simulink model "snap2_f_200msps_64i_4096c"  (R2019a)
settings: Solver=VariableStepDiscrete  StartTime=0.0  StopTime=10.0  RelTol=1e-3
undefined symbols (not defined in the file or in its folder): datetime, posixtime
libraries: xbsIndex_r4 x21354, casper_library_misc x297, casper_library_delays x19, xps_library x14, casper_library_sources x4
(part 2 of 217)

== system snap2_f_200msps_64i_4096c/SNAP2 ==

== system snap2_f_200msps_64i_4096c/aaa_onegbe ==
  Constant : xbsIndex_r4/Constant  const=0  gui_display_data_type=Boolean  arith_type=Boolean  n_bits=16  bin_pt=14  preci_type=Single  exp_width=8  frac_width=24  explicit_period=on  period=1  equ=P=C  opselect=C  inp2=PCIN>>17  opr=+  inp1=P  carry=CIN  dbl_ovrd=off  block_type=constant
  Constant1 : xbsIndex_r4/Constant  const=0  gui_display_data_type=Fixed-point  arith_type=Unsigned  n_bits=8  bin_pt=0  preci_type=Single  exp_width=8  frac_width=24  explicit_period=on  period=1  equ=P=C  opselect=C  inp2=PCIN>>17  opr=+  inp1=P  carry=CIN  dbl_ovrd=off  block_type=constant
  Constant2 : xbsIndex_r4/Constant  const=1  gui_display_data_type=Boolean  arith_type=Boolean  n_bits=16  bin_pt=14  preci_type=Single  exp_width=8  frac_width=24  explicit_period=on  period=1  equ=P=C  opselect=C  inp2=PCIN>>17  opr=+  inp1=P  carry=CIN  dbl_ovrd=off  block_type=constant
  Constant3 : xbsIndex_r4/Constant  const=0  gui_display_data_type=Fixed-point  arith_type=Unsigned  n_bits=32  bin_pt=0  preci_type=Single  exp_width=8  frac_width=24  explicit_period=on  period=1  equ=P=C  opselect=C  inp2=PCIN>>17  opr=+  inp1=P  carry=CIN  dbl_ovrd=off  block_type=constant
  Constant4 : xbsIndex_r4/Constant  const=0  gui_display_data_type=Fixed-point  arith_type=Unsigned  n_bits=16  bin_pt=0  preci_type=Single  exp_width=8  frac_width=24  explicit_period=on  period=1  equ=P=C  opselect=C  inp2=PCIN>>17  opr=+  inp1=P  carry=CIN  dbl_ovrd=off  block_type=constant
  one_GbE : xps_library/IO/one_gbe  Tag=xps:onegbe  local_en=on  dis_cpu_rx=off  dis_cpu_tx=off  cpu_promiscuous=off  local_mac=hex2dec('123456789abc')  local_ip=hex2dec('c0a8290a')  local_port=4321  local_gateway=1
      settings: SourceProductName=CASPER XPS Blockset
  wires:
  Constant/1 -> one_GbE/7, one_GbE/4, one_GbE/2, one_GbE/1
  Constant3/1 -> one_GbE/5
  Constant1/1 -> one_GbE/3
  Constant2/1 -> one_GbE/8
  Constant4/1 -> one_GbE/6

== system snap2_f_200msps_64i_4096c/adc ==
  chip_sync : Inport
  Delay{1..70,72} (71 alike) : xbsIndex_r4/Delay  rst=off  infoeditControl=Selection of Reset will increase slice count due to use of real FFs and instead of SRLs  en=off  latency=1  reg_retiming=off  dbl_ovrd=off  block_type=delay
  Logical : xbsIndex_r4/Logical  logical_function=OR  inputs=2  en=off  latency=1  precision=Full  arith_type=Unsigned  n_bits=16  bin_pt=0  align_bp=on  dbl_ovrd=off  block_type=logical
  Logical1 : xbsIndex_r4/Logical  logical_function=AND  inputs=2  en=off  latency=1  precision=Full  arith_type=Unsigned  n_bits=16  bin_pt=0  align_bp=on  dbl_ovrd=off  block_type=logical
  Logical3 : xbsIndex_r4/Logical  logical_function=OR  inputs=2  en=off  latency=1  precision=Full  arith_type=Unsigned  n_bits=16  bin_pt=0  align_bp=on  dbl_ovrd=off  block_type=logical
  Logical4 : xbsIndex_r4/Logical  logical_function=AND  inputs=2  en=off  latency=1  precision=Full  arith_type=Unsigned  n_bits=16  bin_pt=0  align_bp=on  dbl_ovrd=off  block_type=logical
  bus_create : Subsystem  AncestorBlock=casper_library_flow_control/bus_create  mask(bus_create){inputNum=64}
      mask prompts: inputNum "Number of inputs:"
      mask init:
      | bus_create_init(gcb,...
      |     'inputNum', inputNum);
  fmc0 : Subsystem  Tag=xps:ads5296x4  AncestorBlock=xps_library/ADCs/ads5296x4  mask(ADS5296x4){board_count=2, sample_rate=200, port=0, clockport=1, version=2}
      mask prompts: board_count "Number of quad-chip ADC Boards"; sample_rate "Sample Rate"; port "Which FMC port?"; clockport "Use clock from which FMC board?"; version "Which ADC board version?"
      mask help: 16-input ADC based on the TI ADS5296 chip.
      mask init:
      | % Only board_count is needed by init function
      | ads5296x4_init(gcb, ...
      |     'board_count', board_count);
      mask TypeOptions board_count: 1 | 2 | 3 | 4
  fmc1 : Subsystem  Tag=xps:ads5296x4  AncestorBlock=xps_library/ADCs/ads5296x4  mask(ADS5296x4){board_count=2, sample_rate=200, port=1, clockport=1, version=2}
      mask prompts: board_count "Number of quad-chip ADC Boards"; sample_rate "Sample Rate"; port "Which FMC port?"; clockport "Use clock from which FMC board?"; version "Which ADC board version?"
      mask help: 16-input ADC based on the TI ADS5296 chip.
      mask init:
      | % Only board_count is needed by init function
      | ads5296x4_init(gcb, ...
      |     'board_count', board_count);
      mask TypeOptions board_count: 1 | 2 | 3 | 4
  sync : Subsystem  Tag=xps:sw_reg  AncestorBlock=xps_library/Memory/software_register  mask(swreg){io_dir=From Processor, io_delay=0, init_val=0, sample_period=1, names=[sync ext_sync_enable ss_trig ext_ss_trig_en rst], bitwidths=[1 1 1 1 1], bin_pts=0, arith_types=2, sim_port=on, show_format=on, desc_str=|}
      mask desc_str=|
      | Write ``1`` to bit 0 to this register to assert the ADC's ``sync``
      | input. This input is edge sensitive.
      | Write ``1`` to bit 1 of this register to enable the external sync input.
      mask prompts: io_dir "I/O direction"; io_delay "I/O delay"; init_val "Initial Value"; sample_period "Sample period"; names "Bitfield names [msb...lsb]"; bitwidths "Bitfield widths"; bin_pts "Bitfield binary pts"; arith_types "Bitfield types, ufix=0, fix=1, bool=2"; sim_port "Provide sim input/output?"; show_format "Print format string?"; desc_str "Description"
      mask help: A 32-bit software-accessible register. Can be divided into bitfields of varying widths and types using the fields in the block mask.
      mask init:
      | swreg_init(gcb)
      settings: AttributesFormatString=5 inputs:b,b,b,b,b = 5 bits
      mask TypeOptions io_dir: To Processor | From Processor
      mask Callback io_dir:
      | mask_enables = get_param(gcb, 'MaskEnables');
      | mask_names = get_param(gcb, 'MaskNames');
      | if strcmp(get_param(gcb, 'io_dir'), 'To Processor'),
      |     mask_enables{ismember(mask_names, 'sample_period')} = 'off';
      | else
      |     mask_enables{ismember(mask_names, 'sample_period')} = 'on';
      | end
      | set_param(gcb, 'MaskEnables', mask_enables);
      mask DialogControl ParameterTabVar0 Prompt: Setup
  adc_data : Outport
  adc_sync : Outport  Port=2
  wires:
  fmc0/33(sync_out) -> ?
  bus_create/1(bus_out) -> adc_data/1
  Delay1/1 -> fmc1/33(sync)
  Delay2/1 -> fmc1/34(snapshot_trig)
  Delay3/1 -> fmc1/36(rst)
  Delay4/1 -> fmc0/36(rst)
  Delay5/1 -> fmc0/34(snapshot_trig)
  Delay6/1 -> fmc0/33(sync)
  fmc1/33(sync_out) -> Delay72/1
  Logical1/1 -> Logical/1
  sync/1(in_sync) -> [int_sync]
  sync/2(in_ext_sync_enable) -> [ext_sync_en]
  sync/3(in_ss_trig) -> [ss_trig]
  sync/4(in_ext_ss_trig_en) -> [ext_ss_trig_en]
  sync/5(in_rst) -> [rst]
  [rst] -> Delay4/1
  [rst] -> Delay3/1
  [ext_sync_en] -> Logical1/2
  [int_sync] -> Logical/2
  Logical/1 -> [adc_sync]
  [adc_sync] -> Delay6/1
  [adc_sync] -> Delay1/1
  Logical3/1 -> [adc_ss_trigger]
  [ss_trig] -> Logical3/2
  [ext_ss_trig_en] -> Logical4/2
  chip_sync/1 -> Logical4/1, Logical1/1
  Logical4/1 -> Logical3/1
  [adc_ss_trigger] -> Delay5/1
  [adc_ss_trigger] -> Delay2/1
  fmc0/1(a1) -> Delay7/1
  fmc0/2(a2) -> Delay8/1
  fmc0/3(a3) -> Delay9/1
  fmc0/4(a4) -> Delay10/1
  fmc0/5(b1) -> Delay12/1
  fmc0/6(b2) -> Delay13/1
  fmc0/7(b3) -> Delay14/1
  fmc0/8(b4) -> Delay11/1
  fmc0/9(c1) -> Delay20/1
  fmc0/10(c2) -> Delay21/1
  fmc0/11(c3) -> Delay22/1
  fmc0/12(c4) -> Delay15/1
  fmc0/13(d1) -> Delay17/1
  fmc0/14(d2) -> Delay18/1
  fmc0/15(d3) -> Delay19/1
  fmc0/19(e3) -> Delay38/1
  fmc0/20(e4) -> Delay23/1
  fmc0/22(f2) -> Delay26/1
  fmc0/26(g2) -> Delay34/1
  fmc0/30(h2) -> Delay31/1
  fmc0/25(g1) -> Delay33/1
  fmc0/23(f3) -> Delay27/1
  fmc0/18(e2) -> Delay37/1
  fmc0/24(f4) -> Delay24/1
  fmc0/28(g4) -> Delay28/1
  fmc0/16(d4) -> Delay16/1
  fmc0/27(g3) -> Delay35/1
  fmc0/17(e1) -> Delay36/1
  fmc0/21(f1) -> Delay25/1
  fmc0/29(h1) -> Delay30/1
  fmc1/25(g1) -> Delay65/1
  fmc1/2(a2) -> Delay53/1
  fmc1/10(c2) -> Delay50/1
  fmc1/5(b1) -> Delay41/1
  fmc1/4(a4) -> Delay39/1
  fmc1/12(c4) -> Delay44/1
  fmc1/7(b3) -> Delay43/1
  fmc1/18(e2) -> Delay69/1
  fmc1/22(f2) -> Delay58/1
  fmc1/14(d2) -> Delay47/1
  fmc1/19(e3) -> Delay70/1
  fmc1/17(e1) -> Delay68/1
  fmc1/1(a1) -> Delay52/1
  fmc1/24(f4) -> Delay56/1
  fmc0/31(h3) -> Delay32/1
  fmc1/27(g3) -> Delay67/1
  fmc1/8(b4) -> Delay40/1
  fmc1/15(d3) -> Delay48/1
  fmc1/11(c3) -> Delay51/1
  fmc1/13(d1) -> Delay46/1
  fmc0/32(h4) -> Delay29/1
  fmc1/6(b2) -> Delay42/1
  fmc1/3(a3) -> Delay54/1
  fmc1/16(d4) -> Delay45/1
  fmc1/26(g2) -> Delay66/1
  fmc1/9(c1) -> Delay49/1
  fmc1/21(f1) -> Delay57/1
  fmc1/23(f3) -> Delay59/1
  fmc1/20(e4) -> Delay55/1
  fmc1/28(g4) -> Delay60/1
  fmc1/32(h4) -> Delay61/1
  fmc1/30(h2) -> Delay63/1
  fmc1/31(h3) -> Delay64/1
  fmc1/29(h1) -> Delay62/1
  Delay72/1 -> adc_sync/1
  Delay7/1 -> bus_create/1(in1)
  Delay8/1 -> bus_create/2(in2)
  Delay9/1 -> bus_create/3(in3)
  Delay10/1 -> bus_create/4(in4)
  Delay13/1 -> bus_create/6(in6)
  Delay14/1 -> bus_create/7(in7)
  Delay12/1 -> bus_create/5(in5)
  Delay11/1 -> bus_create/8(in8)
  Delay21/1 -> bus_create/10(in10)
  Delay17/1 -> bus_create/13(in13)
  Delay16/1 -> bus_create/16(in16)
  Delay20/1 -> bus_create/9(in9)
  Delay15/1 -> bus_create/12(in12)
  Delay22/1 -> bus_create/11(in11)
  Delay19/1 -> bus_create/15(in15)
  Delay18/1 -> bus_create/14(in14)
  Delay26/1 -> bus_create/22(in22)
  Delay33/1 -> bus_create/25(in25)
  Delay35/1 -> bus_create/27(in27)
  Delay34/1 -> bus_create/26(in26)
  Delay36/1 -> bus_create/17(in17)
  Delay27/1 -> bus_create/23(in23)
  Delay32/1 -> bus_create/31(in31)
  Delay25/1 -> bus_create/21(in21)
  Delay29/1 -> bus_create/32(in32)
  Delay38/1 -> bus_create/19(in19)
  Delay28/1 -> bus_create/28(in28)
  Delay31/1 -> bus_create/30(in30)
  Delay30/1 -> bus_create/29(in29)
  Delay24/1 -> bus_create/24(in24)
  Delay37/1 -> bus_create/18(in18)
  Delay23/1 -> bus_create/20(in20)
  Delay42/1 -> bus_create/38(in38)
  Delay50/1 -> bus_create/42(in42)
  Delay39/1 -> bus_create/36(in36)
  Delay53/1 -> bus_create/34(in34)
  Delay51/1 -> bus_create/43(in43)
  Delay40/1 -> bus_create/40(in40)
  Delay52/1 -> bus_create/33(in33)
  Delay47/1 -> bus_create/46(in46)
  Delay41/1 -> bus_create/37(in37)
  Delay54/1 -> bus_create/35(in35)
  Delay49/1 -> bus_create/41(in41)
  Delay43/1 -> bus_create/39(in39)
  Delay48/1 -> bus_create/47(in47)
  Delay44/1 -> bus_create/44(in44)
  Delay46/1 -> bus_create/45(in45)
  Delay45/1 -> bus_create/48(in48)
  Delay55/1 -> bus_create/52(in52)
  Delay60/1 -> bus_create/60(in60)
  Delay65/1 -> bus_create/57(in57)
  Delay68/1 -> bus_create/49(in49)
  Delay66/1 -> bus_create/58(in58)
  Delay69/1 -> bus_create/50(in50)
  Delay64/1 -> bus_create/63(in63)
  Delay56/1 -> bus_create/56(in56)
  Delay58/1 -> bus_create/54(in54)
  Delay59/1 -> bus_create/55(in55)
  Delay70/1 -> bus_create/51(in51)
  Delay62/1 -> bus_create/61(in61)
  Delay61/1 -> bus_create/64(in64)
  Delay57/1 -> bus_create/53(in53)
  Delay63/1 -> bus_create/62(in62)
  Delay67/1 -> bus_create/59(in59)

== system snap2_f_200msps_64i_4096c/autocorr ==
  note: acc_len in spectra
  sync : Inport
  din : Inport  Port=2
  rst : Inport  Port=3
  0 : Subsystem  Commented=on  mask{nchan_bits=nchan_bits, npol_bits=npol_bits - 2}
      mask prompts: nchan_bits "Number of channels (2^?)"; npol_bits "Number of pols (2^?)"
  1 : Subsystem  Commented=on  mask{nchan_bits=nchan_bits, npol_bits=npol_bits - 2}
      mask prompts: nchan_bits "Number of channels (2^?)"; npol_bits "Number of pols (2^?)"
  2 : Subsystem  Commented=on  mask{nchan_bits=nchan_bits, npol_bits=npol_bits - 2}
      mask prompts: nchan_bits "Number of channels (2^?)"; npol_bits "Number of pols (2^?)"
  3 : Subsystem  Commented=on  mask{nchan_bits=nchan_bits, npol_bits=npol_bits - 2}
      mask prompts: nchan_bits "Number of channels (2^?)"; npol_bits "Number of pols (2^?)"
  Constant : xbsIndex_r4/Constant  const=0  gui_display_data_type=Fixed-point  arith_type=Unsigned  n_bits=288  bin_pt=0  preci_type=Single  exp_width=8  frac_width=24  explicit_period=on  period=1  equ=P=C  opselect=C  inp2=PCIN>>17  opr=+  inp1=P  carry=CIN  dbl_ovrd=off  block_type=constant
  Constant6 : Constant  Value=1024
  Counter1 : xbsIndex_r4/Counter  cnt_type=Free Running  cnt_to=Inf  operation=Up  start_count=0  cnt_by_val=1  arith_type=Unsigned  n_bits=32  bin_pt=0  load_pin=off  rst=off  en=on  explicit_period=on  period=1  use_behavioral_HDL=off  implementation=Fabric  dbl_ovrd=off  block_type=counter
  Delay1 : xbsIndex_r4/Delay  rst=off  infoeditControl=Selection of Reset will increase slice count due to use of real FFs and instead of SRLs  en=off  latency=1  reg_retiming=on  dbl_ovrd=off  block_type=delay
  Delay2 : xbsIndex_r4/Delay  rst=off  infoeditControl=Selection of Reset will increase slice count due to use of real FFs and instead of SRLs  en=off  latency=1  reg_retiming=on  dbl_ovrd=off  block_type=delay
  Delay3 : xbsIndex_r4/Delay  rst=off  infoeditControl=Selection of Reset will increase slice count due to use of real FFs and instead of SRLs  en=off  latency=3  reg_retiming=on  dbl_ovrd=off  block_type=delay
  From{,2,5,10} (4 alike) : From  Commented=on  GotoTag=sync
  From{1,3,6,11} (4 alike) : From  Commented=on  GotoTag=rst
  From{4,7,9,12} (4 alike) : From  Commented=on  GotoTag=acc_len
  From13 : From  Commented=on  GotoTag=chan16_32
  From14 : From  Commented=on  GotoTag=chan32_48
  From15 : From  Commented=on  GotoTag=chan48_64
  From16 : From  Commented=on  GotoTag=chan0_16
  From{25..28} (4 alike) : From  Commented=on  GotoTag=trig
  Goto2 : Goto  Commented=on  GotoTag=new_acc
  Mux : xbsIndex_r4/Mux  inputs=5  en=off  latency=1  precision=Full  arith_type=Unsigned  n_bits=16  bin_pt=14  quantization=Truncate  overflow=Wrap  dbl_ovrd=off  block_type=mux
  Slice1 : xbsIndex_r4/Slice  nbits=32-nchan_bits-npol_bits  boolean_output=off  mode=Lower Bit Location + Width  bit1=0  base1=MSB of Input  bit0=0  base0=LSB of Input  dbl_ovrd=off  block_type=slice
  acc_cnt : Subsystem  Tag=xps:sw_reg  AncestorBlock=xps_library/Memory/software_register  mask(swreg){io_dir=To Processor, io_delay=0, init_val=0, sample_period=1, names=reg, bitwidths=32, bin_pts=0, arith_types=0, sim_port=on, show_format=on, desc_str=|}
      mask desc_str=|
      | 32-bit wrapping accumulation counter, which increments each
      | time a new accumulation is recorded to RAM.
      | There is no buffer locking when correlation data are
      | read, so this counter can be used to ensure that data
      | have not changed during a read.
      mask prompts: io_dir "I/O direction"; io_delay "I/O delay"; init_val "Initial Value"; sample_period "Sample period"; names "Bitfield names [msb...lsb]"; bitwidths "Bitfield widths"; bin_pts "Bitfield binary pts"; arith_types "Bitfield types, ufix=0, fix=1, bool=2"; sim_port "Provide sim input/output?"; show_format "Print format string?"; desc_str "Description"
      mask help: A 32-bit software-accessible register. Can be divided into bitfields of varying widths and types using the fields in the block mask.
      mask init:
      | swreg_init(gcb)
      settings: AttributesFormatString=1output:uf32.0 = 32 bits
      mask TypeOptions io_dir: To Processor | From Processor
      mask Callback io_dir:
      | mask_enables = get_param(gcb, 'MaskEnables');
      | mask_names = get_param(gcb, 'MaskNames');
      | if strcmp(get_param(gcb, 'io_dir'), 'To Processor'),
      |     mask_enables{ismember(mask_names, 'sample_period')} = 'off';
      | else
      |     mask_enables{ismember(mask_names, 'sample_period')} = 'on';
      | end
      | set_param(gcb, 'MaskEnables', mask_enables);
      mask DialogControl ParameterTabVar0 Prompt: Setup
  acc_len : Subsystem  Tag=xps:sw_reg  AncestorBlock=xps_library/Memory/software_register  mask(swreg){io_dir=From Processor, io_delay=0, init_val=0, sample_period=1, names=reg, bitwidths=32, bin_pts=0, arith_types=0, sim_port=on, show_format=on, desc_str=Accumulation length, in spectra.}
      mask prompts: io_dir "I/O direction"; io_delay "I/O delay"; init_val "Initial Value"; sample_period "Sample period"; names "Bitfield names [msb...lsb]"; bitwidths "Bitfield widths"; bin_pts "Bitfield binary pts"; arith_types "Bitfield types, ufix=0, fix=1, bool=2"; sim_port "Provide sim input/output?"; show_format "Print format string?"; desc_str "Description"
      mask help: A 32-bit software-accessible register. Can be divided into bitfields of varying widths and types using the fields in the block mask.
      mask init:
      | swreg_init(gcb)
      settings: AttributesFormatString=1input:uf32.0 = 32 bits
      mask TypeOptions io_dir: To Processor | From Processor
      mask Callback io_dir:
      | mask_enables = get_param(gcb, 'MaskEnables');
      | mask_names = get_param(gcb, 'MaskNames');
      | if strcmp(get_param(gcb, 'io_dir'), 'To Processor'),
      |     mask_enables{ismember(mask_names, 'sample_period')} = 'off';
      | else
      |     mask_enables{ismember(mask_names, 'sample_period')} = 'on';
      | end
      | set_param(gcb, 'MaskEnables', mask_enables);
      mask DialogControl ParameterTabVar0 Prompt: Setup
  bus_expand : Subsystem  AncestorBlock=casper_library_flow_control/bus_expand  mask(bus_expand){mode=divisions of equal size, outputNum=4, outputWidth=18*2*8, outputBinaryPt=0, outputArithmeticType=0, show_format=off, outputToWorkspace=off, variablePrefix=out, outputToModelAsWell=on}
      mask prompts: outputNum "Number of outputs:"; outputWidth "Output width:"; outputBinaryPt "Output binary point position:"; outputArithmeticType "Output arithmetic type (ufix=0, fix=1, bool=2):"; show_format "Print format string?"; outputToWorkspace "Output to workspace?"; variablePrefix "Variable name prefix:"; outputToModelAsWell "Output to model as well?"
      mask help:
      | Expands a 'bus' made using a bus_create or Xilinx
      | concat block.
      | The input will be divided into the specified number
      | of outputs with the specified arithmetic types.
      | Divisions are made from most significant bit.
      mask init:
      | bus_expand_init(gcb,...
      |     'mode', mode, ...
      |     'outputNum', outputNum, ...
      |     'outputWidth', outputWidth, ...
      |     'outputBinaryPt', outputBinaryPt, ...
      |     'outputArithmeticType', outputArithmeticType, ...
      |     'show_format', show_format, ...
      |     'outputToWorkspace', outputToWorkspace, ...
      |     'variablePrefix', variablePrefix, ...
      |     'outputToModelAsWell', outputToModelAsWell);
      settings: AttributesFormatString=4 outputs
      mask TypeOptions mode: divisions of equal size | divisions of arbitrary size
      mask Callback mode: bus_expand_callback();
      mask Callback outputWidth: bus_expand_callback();
      mask Callback outputToWorkspace: bus_expand_callback();
  common : Subsystem  mask{nchan_bits=nchan_bits, npol_bits=npol_bits - 2}
      mask prompts: nchan_bits "Number of channels (2^?)"; npol_bits "Number of pols (2^?)"
  mux_sel : Subsystem  Tag=xps:sw_reg  AncestorBlock=xps_library/Memory/software_register  mask(swreg){io_dir=From Processor, io_delay=0, init_val=0, sample_period=1, names=reg, bitwidths=3, bin_pts=0, arith_types=0, sim_port=on, show_format=on, desc_str=|}
      mask desc_str=|
      | Input selection controller. Set bits ``[1:0]`` to ``n``
      | to compute the autocorrelations of F-engine inputs
      | ``16n..16(n+1)-1``.
      mask prompts: io_dir "I/O direction"; io_delay "I/O delay"; init_val "Initial Value"; sample_period "Sample period"; names "Bitfield names [msb...lsb]"; bitwidths "Bitfield widths"; bin_pts "Bitfield binary pts"; arith_types "Bitfield types, ufix=0, fix=1, bool=2"; sim_port "Provide sim input/output?"; show_format "Print format string?"; desc_str "Description"
      mask help: A 32-bit software-accessible register. Can be divided into bitfields of varying widths and types using the fields in the block mask.
      mask init:
      | swreg_init(gcb)
      settings: AttributesFormatString=1input:uf3.0 = 3 bits
      mask TypeOptions io_dir: To Processor | From Processor
      mask Callback io_dir:
      | mask_enables = get_param(gcb, 'MaskEnables');
      | mask_names = get_param(gcb, 'MaskNames');
      | if strcmp(get_param(gcb, 'io_dir'), 'To Processor'),
      |     mask_enables{ismember(mask_names, 'sample_period')} = 'off';
      | else
      |     mask_enables{ismember(mask_names, 'sample_period')} = 'on';
      | end
      | set_param(gcb, 'MaskEnables', mask_enables);
      mask DialogControl ParameterTabVar0 Prompt: Setup
  trig : Subsystem  Tag=xps:sw_reg  AncestorBlock=xps_library/Memory/software_register  mask(swreg){io_dir=From Processor, io_delay=0, init_val=0, sample_period=1, names=reg, bitwidths=1, bin_pts=0, arith_types=2, sim_port=on, show_format=on, desc_str="Transition bit 0 from 0 to 1 to trigger a capture of the next valid accumulation"}
      mask prompts: io_dir "I/O direction"; io_delay "I/O delay"; init_val "Initial Value"; sample_period "Sample period"; names "Bitfield names [msb...lsb]"; bitwidths "Bitfield widths"; bin_pts "Bitfield binary pts"; arith_types "Bitfield types, ufix=0, fix=1, bool=2"; sim_port "Provide sim input/output?"; show_format "Print format string?"; desc_str "Description"
      mask help: A 32-bit software-accessible register. Can be divided into bitfields of varying widths and types using the fields in the block mask.
      mask init:
      | swreg_init(gcb)
      settings: AttributesFormatString=1input:b = 1 bits
      mask TypeOptions io_dir: To Processor | From Processor
      mask Callback io_dir:
      | mask_enables = get_param(gcb, 'MaskEnables');
      | mask_names = get_param(gcb, 'MaskNames');
      | if strcmp(get_param(gcb, 'io_dir'), 'To Processor'),
      |     mask_enables{ismember(mask_names, 'sample_period')} = 'off';
      | else
      |     mask_enables{ismember(mask_names, 'sample_period')} = 'on';
      | end
      | set_param(gcb, 'MaskEnables', mask_enables);
      mask DialogControl ParameterTabVar0 Prompt: Setup
  wires:
  din/1 -> bus_expand/1(bus_in)
  sync/1 -> [sync]
  rst/1 -> [rst]
  From/1 -> 0/1(sync)
  From1/1 -> 0/3(rst)
  acc_len/1(in_reg) -> Slice1/1
  Constant6/1 -> acc_len/1(sim_1)
  Slice1/1 -> [acc_len]
  [new_acc] -> Counter1/1
  Delay2/1 -> acc_cnt/1(out_reg)
  Counter1/1 -> Delay2/1
  From9/1 -> 0/4(acc_len)
  From4/1 -> 1/4(acc_len)
  From3/1 -> 1/3(rst)
  From2/1 -> 1/1(sync)
  From5/1 -> 2/1(sync)
  From6/1 -> 2/3(rst)
  From7/1 -> 2/4(acc_len)
  From12/1 -> 3/4(acc_len)
  From11/1 -> 3/3(rst)
  From10/1 -> 3/1(sync)
  bus_expand/1(msb_out4) -> [chan0_16]
  bus_expand/2(out3) -> [chan16_32]
  bus_expand/3(out2) -> [chan32_48]
  bus_expand/4(lsb_out1) -> [chan48_64]
  From13/1 -> 1/2(din)
  From14/1 -> 2/2(din)
  From15/1 -> 3/2(din)
  From16/1 -> 0/2(din)
  Mux/1 -> common/2(din)
  [acc_len] -> common/4(acc_len)
  common/1(new_acc) -> [new_acc]
  [rst] -> common/3(rst)
  [sync] -> Delay1/1
  Delay1/1 -> common/1(sync)
  [chan0_16] -> Mux/2
  mux_sel/1(in_reg) -> Delay3/1
  [chan16_32] -> Mux/3
  [chan32_48] -> Mux/4
  [chan48_64] -> Mux/5
  Delay3/1 -> Mux/1
  [trig] -> common/5(trig)
  trig/1(in_reg) -> [trig]
  From25/1 -> 0/5(trig)
  0/1(new_acc) -> Goto2/1
  From26/1 -> 1/5(trig)
  From27/1 -> 2/5(trig)
  From28/1 -> 3/5(trig)
  Constant/1 -> Mux/6

== system snap2_f_200msps_64i_4096c/chan_reorder ==
  note: manually make
      | runtime configurable
      |
      | NB: allowed sync period
      | is unknown!!
  note: block transpose
      | last two words, so pol order is
      | 0, 1, ..., 31 (first word)
      | 32, 33, ..., 63 (second word)
  note: blockwise transpose:
      |
      | output order is now:
      |
      | chans (512) x pols (2) x chans (8) x pols (32)
      |
      | last axis here is pol:
      | n, n+16, n+32, n+48,
      | n+1, n+17, n+32, n+49, ...
      | ...
      | n+7, n+23, n+39, n+55
  note: Reorder each word:
      |
      | order is now:
      |
      | chans (512) x pols (16) x chans (8) x pols (4)
      |
      | Last index here is pol: n, n+16, n+32, n+48
  note: Input order is:
      |
      | pols (16) x chans (512) x pols (4) x chans (8)
      |
      | Transpose first two axes. Output order is:
      | chans (512) x pols (16) x pols (4) x chans (8)
  note: Use this programmable
      | map to mess with the channel
      | ordering.
      |
      | Out of every block of 128 channels,
      | only the first 80 will be sent.
      | So fold the edges of the band into unwanted slots
      |
      | Input is 8 channels x 4 antennas in parallel.
      | Over 512 clocks we get a full spectrum for these 4 antennas.
      | Over the next 16x512 clocks we get spectra for 64 antennas total
  note: Serial transpose along fastest axes
      |
      | output order is now:
      |
      | chans (512) x chans (8) x pols (2) x pols (32)
  sync : Inport
  din : Inport  Port=2
  Constant : xbsIndex_r4/Constant  const=1  gui_display_data_type=Boolean  arith_type=Boolean  n_bits=1  bin_pt=0  preci_type=Single  exp_width=8  frac_width=24  explicit_period=on  period=1  equ=P=C  opselect=C  inp2=PCIN>>17  opr=+  inp1=P  carry=CIN  dbl_ovrd=off  block_type=constant
  Constant2 : xbsIndex_r4/Constant  const=1  gui_display_data_type=Boolean  arith_type=Boolean  n_bits=1  bin_pt=0  preci_type=Single  exp_width=8  frac_width=24  explicit_period=on  period=1  equ=P=C  opselect=C  inp2=PCIN>>17  opr=+  inp1=P  carry=CIN  dbl_ovrd=off  block_type=constant
  Constant3 : xbsIndex_r4/Constant  const=1  gui_display_data_type=Boolean  arith_type=Boolean  n_bits=1  bin_pt=0  preci_type=Single  exp_width=8  frac_width=24  explicit_period=on  period=1  equ=P=C  opselect=C  inp2=PCIN>>17  opr=+  inp1=P  carry=CIN  dbl_ovrd=off  block_type=constant
  Gateway Out{1..8} (8 alike) : xbsIndex_r4/Gateway Out  inherit_from_input=off  hdl_port=off  rows=1  columns=1  UseAsDAC=off  DACChannel='1'  interface=None  automatic_assignment=on  address_offset=hex2dec('00')  intf_name=''  intf_description=''  timing_constraint=None  locs_specified=off  LOCs={}  io_standard={}  block_type=gatewayout
  Scope{,1..3} (4 alike) : Scope  NumInputPorts=3
  Slice{1..4} (4 alike) : xbsIndex_r4/Slice  nbits=8  boolean_output=off  mode=Lower Bit Location + Width  bit1=9  base1=MSB of Input  bit0=256-8  base0=LSB of Input  dbl_ovrd=off  block_type=slice
  bus_create : Subsystem  AncestorBlock=casper_library_flow_control/bus_create  mask(bus_create){inputNum=8}
      mask prompts: inputNum "Number of inputs:"
      mask init:
      | bus_create_init(gcb,...
      |     'inputNum', inputNum);
  bus_expand2 : Subsystem  AncestorBlock=casper_library_flow_control/bus_expand  mask(bus_expand){mode=divisions of equal size, outputNum=8, outputWidth=4*8, outputBinaryPt=0, outputArithmeticType=0, show_format=off, outputToWorkspace=off, variablePrefix=out, outputToModelAsWell=on}
      mask prompts: outputNum "Number of outputs:"; outputWidth "Output width:"; outputBinaryPt "Output binary point position:"; outputArithmeticType "Output arithmetic type (ufix=0, fix=1, bool=2):"; show_format "Print format string?"; outputToWorkspace "Output to workspace?"; variablePrefix "Variable name prefix:"; outputToModelAsWell "Output to model as well?"
      mask help:
      | Expands a 'bus' made using a bus_create or Xilinx
      | concat block.
      | The input will be divided into the specified number
      | of outputs with the specified arithmetic types.
      | Divisions are made from most significant bit.
      mask init: same as snap2_f_200msps_64i_4096c/autocorr/bus_expand
      settings: AttributesFormatString=8 outputs
      mask TypeOptions mode: divisions of equal size | divisions of arbitrary size
      mask Callback mode: bus_expand_callback();
      mask Callback outputWidth: bus_expand_callback();
      mask Callback outputToWorkspace: bus_expand_callback();
  dynamic : Subsystem  AncestorBlock=casper_library_reorder/reorder  mask(reorder){map=reshape(reshape([0:512 - 1], 256, 2)', 1, 512), n_bits=32*8, n_inputs=1, bram_latency=3, map_latency=3, fanout_latency=0, double_buffer=0, bram_map=on, software_controlled=off}
      mask prompts: map "Output Order:"; n_bits "Data width in"; n_inputs "Number of inputs"; bram_latency "BRAM Latency"; map_latency "Map Latency"; fanout_latency "Fanout latency"; double_buffer "Double Buffer"; bram_map "Use BlockRAM for Map"; software_controlled "Use runtime software control"
      mask init:
      | reorder_init(gcb, ...
      |     'map', map, ...
      |     'n_bits', n_bits, ...
      |     'n_inputs', n_inputs, ...
      |     'bram_latency', bram_latency, ...
      |     'map_latency', map_latency, ...
      |     'fanout_latency', fanout_latency, ...
      |     'double_buffer', double_buffer, ...
      |     'bram_map', bram_map, ...
      |     'software_controlled', software_controlled);
      settings: AttributesFormatString=order=9
      mask Help: eval('xlWeb(''http://casper.berkeley.edu/wiki/Reorder'')')
  parallel_reorder : Subsystem
  pol_reorder : Subsystem
  reorder : Subsystem  AncestorBlock=casper_library_reorder/reorder  mask(reorder){map=reshape(reshape([0:8192 - 1], 512, 16)', 1, 8192), n_bits=8*4*8, n_inputs=1, bram_latency=3, map_latency=1, fanout_latency=0, double_buffer=0, bram_map=on, software_controlled=off}
      mask prompts: map "Output Order:"; n_bits "Data width in"; n_inputs "Number of inputs"; bram_latency "BRAM Latency"; map_latency "Map Latency"; fanout_latency "Fanout latency"; double_buffer "Double Buffer"; bram_map "Use BlockRAM for Map"; software_controlled "Use runtime software control"
      mask init: same as snap2_f_200msps_64i_4096c/chan_reorder/dynamic
      settings: AttributesFormatString=order=13
      mask Help: eval('xlWeb(''http://casper.berkeley.edu/wiki/Reorder'')')
  reorder2 : Subsystem  AncestorBlock=casper_library_reorder/reorder  mask(reorder){map=reshape(reshape([0:16 - 1], 8, 2)', 1, 16), n_bits=32*8, n_inputs=1, bram_latency=3, map_latency=1, fanout_latency=0, double_buffer=0, bram_map=off, software_controlled=off}
      mask prompts: map "Output Order:"; n_bits "Data width in"; n_inputs "Number of inputs"; bram_latency "BRAM Latency"; map_latency "Map Latency"; fanout_latency "Fanout latency"; double_buffer "Double Buffer"; bram_map "Use BlockRAM for Map"; software_controlled "Use runtime software control"
      mask init: same as snap2_f_200msps_64i_4096c/chan_reorder/dynamic
      settings: AttributesFormatString=order=4
      mask Help: eval('xlWeb(''http://casper.berkeley.edu/wiki/Reorder'')')
  square_transposer : Subsystem  AncestorBlock=casper_library_reorder/square_transposer  mask(square_transposer){n_inputs=3, async=off}
      mask prompts: n_inputs "Number of inputs (2^?):"; async "Aynchronus operation"
      mask init:
      | square_transposer_init(gcb,...
      |     'n_inputs', n_inputs, ...
      |     'async', async);
      settings: AttributesFormatString=n_inputs=3
      mask Help: eval('xlWeb(''http://casper.berkeley.edu/wiki/Square_transposer'')')
  sync_out : Outport
  dout : Outport  Port=2
  wires:
  Constant/1 -> reorder/2(en)
  reorder/3(dout0) -> parallel_reorder/1(din)
  Constant2/1 -> dynamic/2(en)
  sync/1 -> dynamic/1(sync)
  din/1 -> dynamic/3(din0)
  dynamic/2(valid) -> ?
  dynamic/3(dout0) -> Slice3/1, reorder/3(din0)
  parallel_reorder/1(dout) -> Slice1/1, bus_expand2/1(bus_in)
  reorder/1(sync_out) -> Gateway Out2/1, square_transposer/1(sync)
  bus_expand2/4(out5) -> square_transposer/5(in3)
  bus_expand2/7(out2) -> square_transposer/8(in6)
  bus_expand2/1(msb_out8) -> square_transposer/2(in0)
  bus_expand2/2(out7) -> square_transposer/3(in1)
  bus_expand2/6(out3) -> square_transposer/7(in5)
  bus_expand2/3(out6) -> square_transposer/4(in2)
  bus_expand2/5(out4) -> square_transposer/6(in4)
  bus_expand2/8(lsb_out1) -> square_transposer/9(in7)
  square_transposer/9(out7) -> bus_create/8(in8)
  square_transposer/8(out6) -> bus_create/7(in7)
  square_transposer/6(out4) -> bus_create/5(in5)
  square_transposer/7(out5) -> bus_create/6(in6)
  square_transposer/2(out0) -> bus_create/1(in1)
  square_transposer/3(out1) -> bus_create/2(in2)
  square_transposer/4(out2) -> bus_create/3(in3)
  square_transposer/5(out3) -> bus_create/4(in4)
  Constant3/1 -> reorder2/2(en)
  bus_create/1(bus_out) -> Slice2/1, reorder2/3(din0)
  reorder2/1(sync_out) -> Gateway Out7/1, pol_reorder/1(sync)
  reorder2/3(dout0) -> Slice4/1, pol_reorder/2(din)
  pol_reorder/1(sync_out) -> sync_out/1
  pol_reorder/2(dout) -> dout/1
  Gateway Out7/1 -> Scope/1
  Gateway Out8/1 -> Scope/2
  Slice4/1 -> Gateway Out8/1
  Slice1/1 -> Gateway Out3/1
  Gateway Out3/1 -> Scope1/2
  Gateway Out2/1 -> Scope1/1
  Gateway Out4/1 -> Scope2/1
  Gateway Out5/1 -> Scope2/2
  Slice2/1 -> Gateway Out5/1
  square_transposer/1(sync_out) -> Gateway Out4/1, reorder2/1(sync)
  Gateway Out6/1 -> Scope3/1
  Gateway Out1/1 -> Scope3/2
  Slice3/1 -> Gateway Out1/1
  dynamic/1(sync_out) -> Gateway Out6/1, reorder/1(sync)

== system snap2_f_200msps_64i_4096c/corr ==
  sync : Inport
  din : Inport  Port=2
  0 : Subsystem  mask{nchan_bits=12, npol_bits=4}
      mask prompts: nchan_bits "Number of channels (2^?)"; npol_bits "Number of pols (2^?)"
  wires:
  sync/1 -> 0/1(sync)
  din/1 -> 0/2(din)
